simulink model "Model_plane"  (R2021b)
settings: Solver=VariableStepAuto  StartTime=0.0  StopTime=10.0  RelTol=1e-3
values from neighbouring files (symbols this model uses):
  P = [9088 7396 6783 5000 4000]    [Table1.m]
undefined symbols (not defined in the file or in its folder): g, gama, m, psi, Psi0, R, teta, Teta0, V0, x0, y0, z0
settings Model: Creator=Анастасия  LastModifiedBy=Анастасия
settings DebuggingCC: UnconnectedInputMsg=none  UnconnectedOutputMsg=none  UnconnectedLineMsg=none
settings ModelReferenceCC: EnableRefExpFcnMdlSchedulingChecks=off
settings RTWCC: GPUComputeCapability=5.0  DLArmComputeVersion=20.02.1

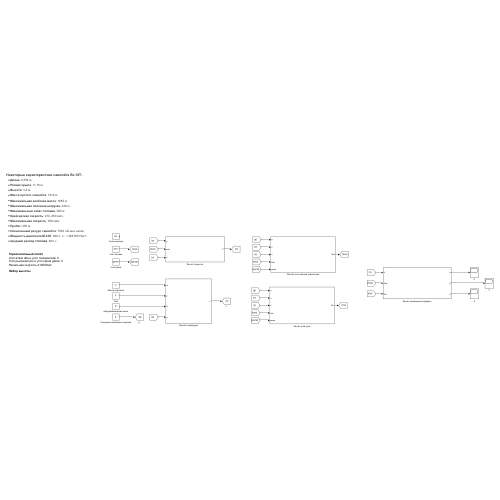
[thumbnail: Simulink's stored preview of the top-level diagram]
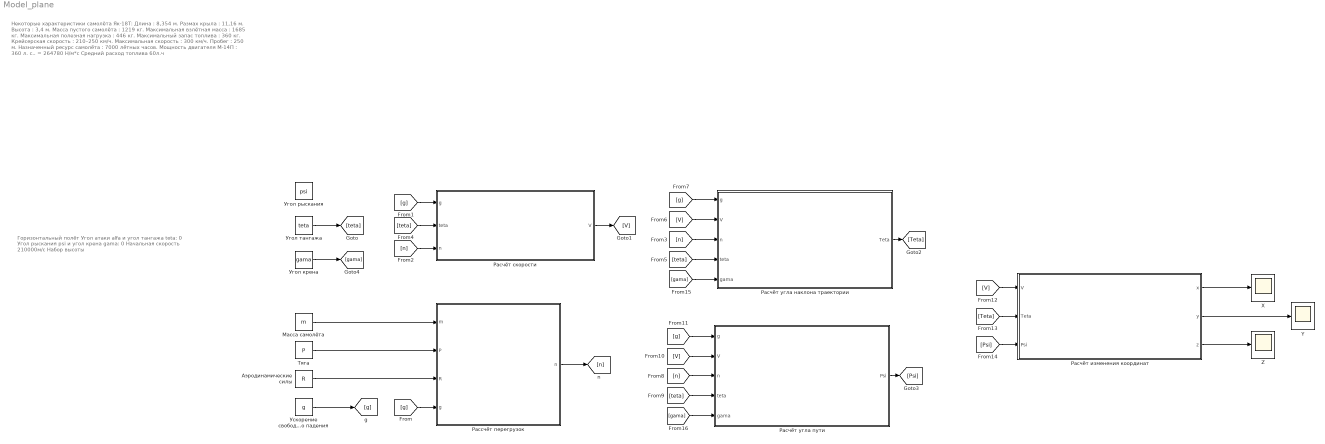
== system Model_plane ==
  note: Горизонтальный полёт
      | Угол атаки alfa и угол тангажа teta: 0
      | Угол рыскания psi и угол крена gama: 0
      | Начальная скорость 210000м/c
      |
      | Набор высоты
  note: Некоторые характеристики самолёта Як-18Т:
      | Длина : 8,354 м.
      | Размах крыла : 11,16 м.
      | Высота : 3,4 м.
      | Масса пустого самолёта : 1219 кг.
      | Максимальная взлётная масса : 1685 кг.
      | Максимальная полезная нагрузка : 446 кг.
      | Максимальный запас топлива : 360 кг.
      | Крейсерская скорость : 210–250 км/ч.
      | Максимальная скорость : 300 км/ч.
      | Пробег : 250 м.
      | Назначенный ресурс самолёта : 7000 лётных часов.
      | Мощность двигателя М-14П : 360 л. с.. = 264780 Н/м*с
      | Средний расход топлива 60л.ч
  X : Scope
  Y : Scope
  Z : Scope
  Аэродинамические силы : Constant  Value=R
  Масса самолёта : Constant  Value=m
  Рассчёт перегрузок : Subsystem
  Расчёт изменения координат : Subsystem
  Расчёт скорости : Subsystem
  Расчёт угла наклона траектории : Subsystem
  Расчёт угла пути : Subsystem
  Тяга : Constant  Value=P
  Угол крена : Constant  Value=gama
  Угол рыскания : Constant  Value=psi
  Угол тангажа : Constant  Value=teta
  Ускорение свободного падения : Constant  Value=g
  wires:
  Тяга/1 -> Рассчёт перегрузок/2(P)
  Аэродинамические силы/1 -> Рассчёт перегрузок/3(R)
  Масса самолёта/1 -> Рассчёт перегрузок/1(m)
  Ускорение свободного падения/1 -> [g]
  [g] -> Рассчёт перегрузок/4(g)
  [g] -> Расчёт скорости/1(g)
  Угол тангажа/1 -> [teta]
  Рассчёт перегрузок/1(n) -> [n]
  [n] -> Расчёт скорости/3(n)
  [n] -> Расчёт угла наклона траектории/3(n)
  [teta] -> Расчёт скорости/2(teta)
  [teta] -> Расчёт угла наклона траектории/4(teta)
  Расчёт скорости/1(V) -> [V]
  [V] -> Расчёт угла наклона траектории/2(V)
  [g] -> Расчёт угла наклона траектории/1(g)
  Расчёт угла наклона траектории/1(Teta) -> [Teta]
  [g] -> Расчёт угла пути/1(g)
  [teta] -> Расчёт угла пути/4(teta)
  Расчёт угла пути/1(Psi) -> [Psi]
  [n] -> Расчёт угла пути/3(n)
  [V] -> Расчёт угла пути/2(V)
  [V] -> Расчёт изменения координат/1(V)
  [Psi] -> Расчёт изменения координат/3(Psi)
  [Teta] -> Расчёт изменения координат/2(Teta)
  Расчёт изменения координат/1(x) -> X/1
  Расчёт изменения координат/2(y) -> Y/1
  Расчёт изменения координат/3(z) -> Z/1
  Угол крена/1 -> [gama]
  [gama] -> Расчёт угла наклона траектории/5(gama)
  [gama] -> Расчёт угла пути/5(gama)

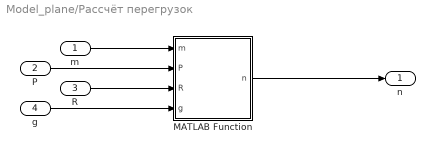
== system Model_plane/Рассчёт перегрузок ==
  m : Inport
  P : Inport  Port=2
  R : Inport  Port=3
  g : Inport  Port=4
  MATLAB Function : MATLAB Function  TreatAsAtomicUnit=on
  n : Outport
  wires:
  g/1 -> MATLAB Function/4(g)
  P/1 -> MATLAB Function/2(P)
  m/1 -> MATLAB Function/1(m)
  R/1 -> MATLAB Function/3(R)
  MATLAB Function/1(n) -> n/1

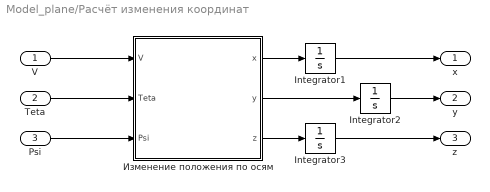
== system Model_plane/Расчёт изменения координат ==
  V : Inport
  Teta : Inport  Port=2
  Psi : Inport  Port=3
  Integrator1 : Integrator  InitialCondition=x0
  Integrator2 : Integrator  InitialCondition=y0
  Integrator3 : Integrator  InitialCondition=z0
  "Изменение положения по осям " : MATLAB Function  TreatAsAtomicUnit=on
  x : Outport
  y : Outport  Port=2
  z : Outport  Port=3
  wires:
  "Изменение положения по осям "/1(x) -> Integrator1/1
  Integrator1/1 -> x/1
  Teta/1 -> "Изменение положения по осям "/2(Teta)
  V/1 -> "Изменение положения по осям "/1(V)
  Psi/1 -> "Изменение положения по осям "/3(Psi)
  "Изменение положения по осям "/2(y) -> Integrator2/1
  Integrator2/1 -> y/1
  "Изменение положения по осям "/3(z) -> Integrator3/1
  Integrator3/1 -> z/1

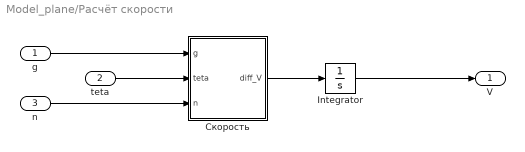
== system Model_plane/Расчёт скорости ==
  g : Inport
  teta : Inport  Port=2
  n : Inport  Port=3
  Integrator : Integrator  InitialCondition=V0
  "Скорость " : MATLAB Function  TreatAsAtomicUnit=on
  V : Outport
  wires:
  g/1 -> "Скорость "/1(g)
  n/1 -> "Скорость "/3(n)
  teta/1 -> "Скорость "/2(teta)
  Integrator/1 -> V/1
  "Скорость "/1(diff_V) -> Integrator/1

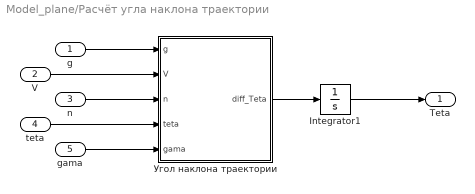
== system Model_plane/Расчёт угла наклона траектории ==
  g : Inport
  V : Inport  Port=2
  n : Inport  Port=3
  teta : Inport  Port=4
  gama : Inport  Port=5
  Integrator1 : Integrator  InitialCondition=Teta0
  "Угол наклона траектории " : MATLAB Function  TreatAsAtomicUnit=on
  Teta : Outport
  wires:
  "Угол наклона траектории "/1(diff_Teta) -> Integrator1/1
  Integrator1/1 -> Teta/1
  g/1 -> "Угол наклона траектории "/1(g)
  V/1 -> "Угол наклона траектории "/2(V)
  n/1 -> "Угол наклона траектории "/3(n)
  teta/1 -> "Угол наклона траектории "/4(teta)
  gama/1 -> "Угол наклона траектории "/5(gama)

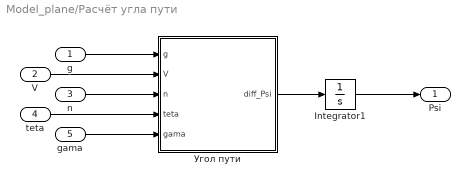
== system Model_plane/Расчёт угла пути ==
  g : Inport
  V : Inport  Port=2
  n : Inport  Port=3
  teta : Inport  Port=4
  gama : Inport  Port=5
  Integrator1 : Integrator  InitialCondition=Psi0
  "Угол пути " : MATLAB Function  TreatAsAtomicUnit=on
  Psi : Outport
  wires:
  "Угол пути "/1(diff_Psi) -> Integrator1/1
  Integrator1/1 -> Psi/1
  g/1 -> "Угол пути "/1(g)
  V/1 -> "Угол пути "/2(V)
  n/1 -> "Угол пути "/3(n)
  teta/1 -> "Угол пути "/4(teta)
  gama/1 -> "Угол пути "/5(gama)

== matlab function Model_plane/Расчёт скорости/Скорость  ==
  data: g input; teta input; n input; diff_V output
function diff_V = fcn(g,teta,n)
    diff_V= g*(n(1)-sin(teta)); 
end

== matlab function Model_plane/Расчёт угла пути/Угол пути  ==
  data: g input; V input; n input; teta input; gama input; diff_Psi output
function diff_Psi = fcn(g,V,n,teta,gama)
    
    diff_Psi= -(g*n(2)*sin(gama))/(V*cos(teta));
    
end

== matlab function Model_plane/Расчёт изменения координат/Изменение положения по осям  ==
  data: V input; Teta input; Psi input; x output; y output; z output
function [x,y,z] = fcn(V, Teta, Psi)
    
    x= V*cos(Teta)*cos(Psi);
    y= V*sin(Teta);
    z= -V*cos(Teta)*sin(Psi);
end

== matlab function Model_plane/Расчёт угла наклона траектории/Угол наклона траектории  ==
  data: g input; V input; n input; teta input; gama input; diff_Teta output
function diff_Teta = fcn(g,V,n,teta, gama)
    
    diff_Teta=(g*(n(2)*cos(gama)-cos(teta)))/V;
    
end

== matlab function Model_plane/Рассчёт перегрузок/MATLAB Function ==
  data: m input; P input; R input; g input; n output
function n = fcn(m,P,R,g)
    alfa=0;  %угол атаки
    beta=0;  %угол скольжения
    fip=180; %угол между тягой силовой установки Р и положительным направлением оси ОХ

    nx = (P*cos(alfa+fip)*cos(beta)-R(1))/(m*g);
    ny = (P*sin(alfa+fip)+R(2))/(m*g);
    nz = (-P*cos(alfa+fip)*sin(beta)+R(3))/(m*g);
    n = [nx,ny,nz];

end
